simulink model "Farmakodynamika"  (R2022b)
settings: Solver=FixedStepAuto  StartTime=0.0  StopTime=1440  FixedStep=1  RelTol=1e-3
values from neighbouring files (symbols this model uses):
  Ag = 0.95    [param1.m]
  Gb = 153    [param1.m]
  ki = 0.1629    [param1.m]
  p2 = best_ch(1,end)    [param1.m]
  Sg = Pop(i,2)    [fitness_last.m]    (also in param1.m = 0.03376)
  Si = best_ch(2,end)    [param1.m]
  Td = Pop(i,1)    [fitness_last.m]    (also in param1.m = 39)
  Ti = 45.383    [param1.m]
  vb = load("Dat_D00_Basal.csv")    [param1.m]
  Vg = 1.467    [param1.m]
  Vi = 139.094    [param1.m]
libraries: dspsigops x1
settings Model: Creator=DFUNDO  LastModifiedBy=DFUNDO

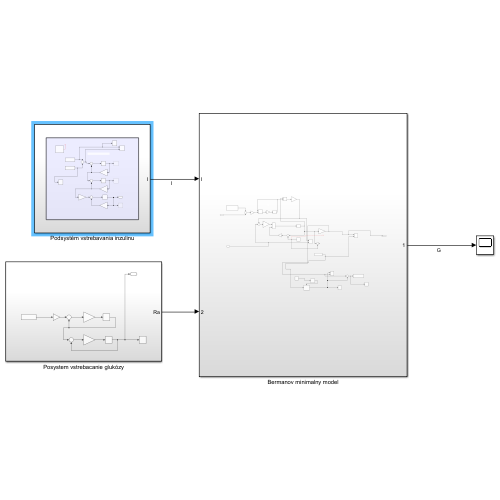
[thumbnail: Simulink's stored preview of the top-level diagram]
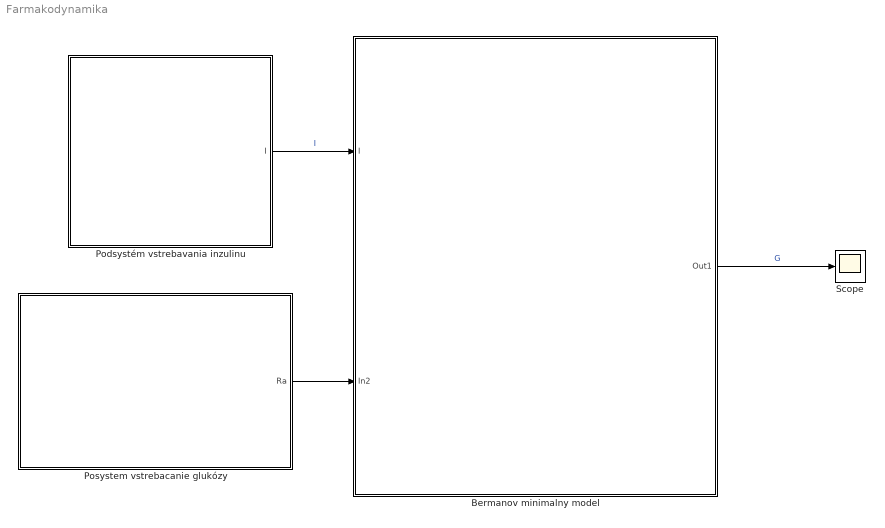
== system Farmakodynamika ==
  Bermanov minimalny model : Subsystem
  Podsystém vstrebavania inzulinu : Subsystem
  Posystem vstrebacanie glukózy : Subsystem
  Scope : Scope
  wires:
  Podsystém vstrebavania inzulinu/1(I) -> Bermanov minimalny model/1(I)  "I"
  Posystem vstrebacanie glukózy/1(Ra) -> Bermanov minimalny model/2(In2)
  Bermanov minimalny model/1(Out1) -> Scope/1  "G"

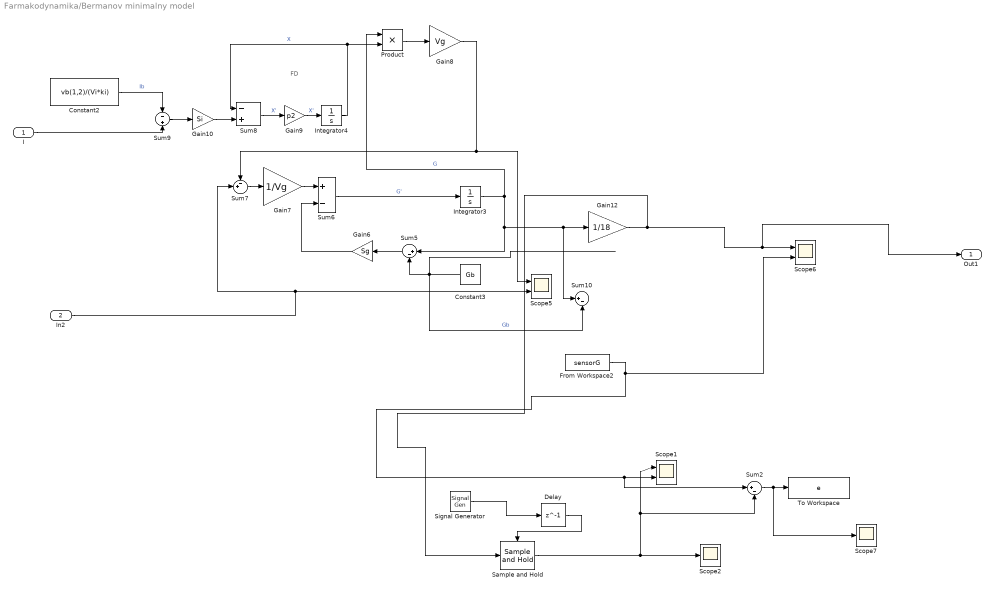
== system Farmakodynamika/Bermanov minimalny model ==
  note: FD
  I : Inport
  In2 : Inport  Port=2
  Constant2 : Constant  Value=vb(1,2)/(Vi*ki)
  Constant3 : Constant  Value=Gb
  Delay : Delay  DelayLength=1
  From Workspace2 : FromWorkspace  VariableName=sensorG  Interpolate=off  OutputAfterFinalValue=Holding final value
  Gain10 : Gain  Gain=Si
  Gain12 : Gain  Gain=1/18
  Gain6 : Gain  Gain=Sg
  Gain7 : Gain  Gain=1/Vg
  Gain8 : Gain  Gain=Vg
  Gain9 : Gain  Gain=p2
  Integrator3 : Integrator  InitialCondition=Gb
  Integrator4 : Integrator
  Product : Product
  Sample and Hold : dspsigops/Sample and Hold  trig=Falling edge  initCond=0  latchinput=off
  Scope1 : Scope  NumInputPorts=2
  Scope2 : Scope
  Scope5 : Scope  NumInputPorts=2
  Scope6 : Scope  NumInputPorts=2
  Scope7 : Scope
  Signal Generator : SignalGenerator  WaveForm=square  Frequency=1/5
  Sum10 : Sum  Inputs=|+-
  Sum2 : Sum  Inputs=|+-
  Sum5 : Sum  Inputs=|+-
  Sum6 : Sum  Inputs=+-
  Sum7 : Sum  Inputs=-+|
  Sum8 : Sum  Inputs=-+
  Sum9 : Sum  Inputs=-+
  To Workspace : ToWorkspace  VariableName=e  SampleTime=-1
      settings: Save2DSignal=2-D array (concatenate along first dimension)
  Out1 : Outport
  wires:
  Sample and Hold/1 -> Scope2/1, Sum2/2, Scope1/1
  From Workspace2/1 -> Sum2/1, Scope1/2, Scope6/2
  Gain12/1 -> Sample and Hold/1, Out1/1, Scope6/1
  Gain10/1 -> Sum8/2
  Integrator3/1 -> Product/1, Sum5/1, Sum10/1, Gain12/1  "G"
  Sum9/1 -> Gain10/1
  Sum5/1 -> Gain6/1
  Gain6/1 -> Sum6/2
  Constant3/1 -> Sum10/2, Sum5/2  "Gb"
  In2/1 -> Sum7/2, Scope5/2
  Sum2/1 -> Scope7/1, To Workspace/1
  Sum6/1 -> Integrator3/1  "G'"
  Integrator4/1 -> Product/2, Sum8/1  "X"
  Sum8/1 -> Gain9/1  "X'"
  Product/1 -> Gain8/1
  Gain9/1 -> Integrator4/1  "X'"
  Sum7/1 -> Gain7/1
  Gain7/1 -> Sum6/1
  Signal Generator/1 -> Delay/1
  Constant2/1 -> Sum9/1  "Ib"
  Gain8/1 -> Sum7/1, Scope5/1
  Delay/1 -> Sample and Hold/Trigger
  I/1 -> Sum9/2

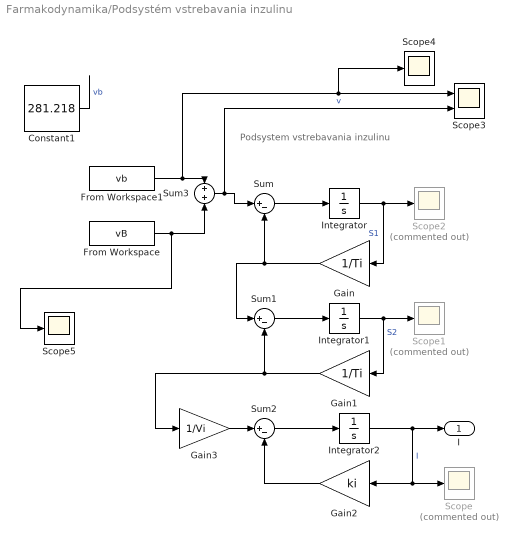
== system Farmakodynamika/Podsystém vstrebavania inzulinu ==
  note: Podsystem vstrebavania inzulinu
  Constant1 : Constant  Value=281.218
  From Workspace : FromWorkspace  VariableName=vB  SampleTime=1  Interpolate=off  ZeroCross=off  OutputAfterFinalValue=Setting to zero
  From Workspace1 : FromWorkspace  VariableName=vb  SampleTime=1  Interpolate=off  ZeroCross=off  OutputAfterFinalValue=Holding final value
  Gain : Gain  Gain=1/Ti
  Gain1 : Gain  Gain=1/Ti
  Gain2 : Gain  Gain=ki
  Gain3 : Gain  Gain=1/Vi
  Integrator : Integrator  InitialCondition=Ti*vb(1,2)
  Integrator1 : Integrator  InitialCondition=Ti*vb(1,2)
  Integrator2 : Integrator  InitialCondition=vb(1,2)/(Vi*ki)
  Scope : Scope  Commented=on
  Scope1 : Scope  Commented=on
  Scope2 : Scope  Commented=on
  Scope3 : Scope  NumInputPorts=2
  Scope4 : Scope
  Scope5 : Scope
  Sum : Sum  Inputs=|+-
  Sum1 : Sum  Inputs=|+-
  Sum2 : Sum  Inputs=|+-
  Sum3 : Sum
  I : Outport
  wires:
  Gain2/1 -> Sum2/2
  Integrator1/1 -> Scope1/1, Gain1/1  "S2"
  Gain/1 -> Sum/2, Sum1/1
  Sum2/1 -> Integrator2/1
  Sum1/1 -> Integrator1/1
  Sum3/1 -> Scope3/2, Sum/1  "v"
  Integrator/1 -> Gain/1, Scope2/1  "S1"
  Gain1/1 -> Gain3/1, Sum1/2
  Gain3/1 -> Sum2/1
  Constant1/1 -> ?  "vb"
  Integrator2/1 -> Gain2/1, Scope/1, I/1  "I"
  Sum/1 -> Integrator/1
  From Workspace/1 -> Scope5/1, Sum3/2
  From Workspace1/1 -> Scope4/1, Scope3/1, Sum3/1

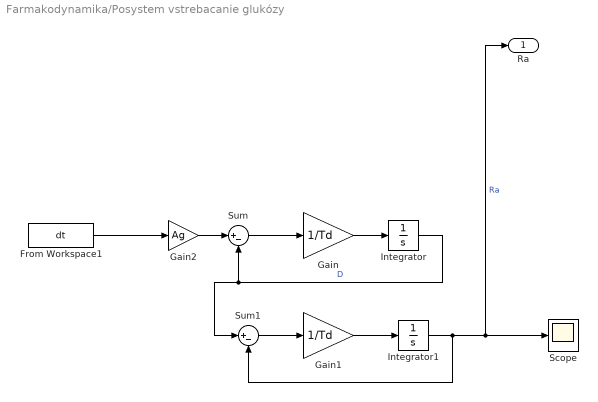
== system Farmakodynamika/Posystem vstrebacanie glukózy ==
  From Workspace1 : FromWorkspace  VariableName=dt  Interpolate=off  OutputAfterFinalValue=Holding final value
  Gain : Gain  Gain=1/Td
  Gain1 : Gain  Gain=1/Td
  Gain2 : Gain  Gain=Ag
  Integrator : Integrator
  Integrator1 : Integrator
  Scope : Scope
  Sum : Sum  Inputs=|+-
  Sum1 : Sum  Inputs=|+-
  Ra : Outport
  wires:
  Integrator1/1 -> Sum1/2, Ra/1, Scope/1  "Ra"
  From Workspace1/1 -> Gain2/1
  Gain/1 -> Integrator/1
  Gain1/1 -> Integrator1/1
  Sum1/1 -> Gain1/1
  Sum/1 -> Gain/1
  Integrator/1 -> Sum1/1, Sum/2  "D"
  Gain2/1 -> Sum/1
